simulink model "DecisionLogic_Stub"  (R2026a)
settings: Solver=VariableStepAuto
settings Model: Creator=HP  LastModifiedBy=HP

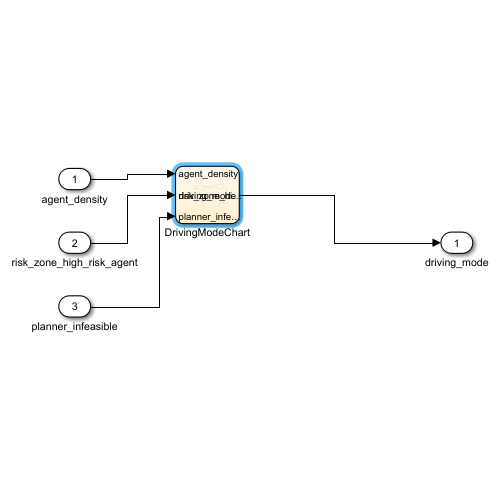
[thumbnail: Simulink's stored preview of the top-level diagram]
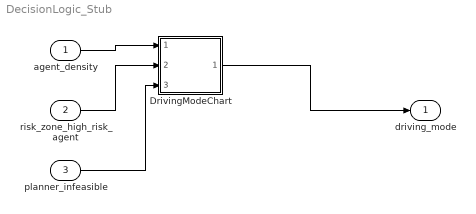
== system DecisionLogic_Stub ==
  agent_density : Inport
  risk_zone_high_risk_agent : Inport  Port=2
  planner_infeasible : Inport  Port=3
  DrivingModeChart : Stateflow chart  TreatAsAtomicUnit=on
  driving_mode : Outport
  wires:
  agent_density/1 -> DrivingModeChart/1(agent_density)
  risk_zone_high_risk_agent/1 -> DrivingModeChart/2(risk_zone_high_risk_agent)
  planner_infeasible/1 -> DrivingModeChart/3(planner_infeasible)
  DrivingModeChart/1(driving_mode) -> driving_mode/1

== stateflow chart DecisionLogic_Stub/DrivingModeChart ==
  state CAUTIOUS
    entry: driving_mode = DrivingMode.CAUTIOUS;
  state CRUISE
    entry: driving_mode = DrivingMode.CRUISE;
  state STOP
    entry: driving_mode = DrivingMode.STOP;
  state YIELD
    entry: driving_mode = DrivingMode.YIELD;
  (default) -> CRUISE
  CAUTIOUS -> STOP [order 3] : [planner_infeasible]
  CRUISE -> YIELD [order 2] : [risk_zone_high_risk_agent]
  YIELD -> CAUTIOUS [order 1] : [~risk_zone_high_risk_agent]
  CRUISE -> CAUTIOUS [order 1] : [agent_density > 3]
  CAUTIOUS -> YIELD [order 2] : [risk_zone_high_risk_agent]
  CAUTIOUS -> CRUISE [order 1] : [agent_density < 1.5]
  STOP -> CRUISE : [~planner_infeasible] % PLACEHOLDER -- confirm recovery semantics with M3/M4
  CRUISE -> STOP [order 3] : [planner_infeasible]
  YIELD -> STOP [order 2] : [planner_infeasible]
  data: agent_density input double; risk_zone_high_risk_agent input boolean; planner_infeasible input boolean; driving_mode output DrivingMode
